simulink model "boostconverter_nap"  (R2016a)
settings: Solver=FixedStepDiscrete  SolverMode=SingleTasking  StartTime=0.0  StopTime=5e-5  FixedStep=5e-5  RelTol=1e-3
PreLoadFcn:
  | waijung.modelPreload; % Required for working with Waijung Blockset. Do not remove.
undefined symbols (not defined in the file): ARM, HSEOSC, Link, LQFP100, MDK, ST, STM32F407VE
libraries: stm32f4_adc_lib x1, stm32f4_device_config_lib x1, stm32f4_tim_lib x1
(part 3 of 3)

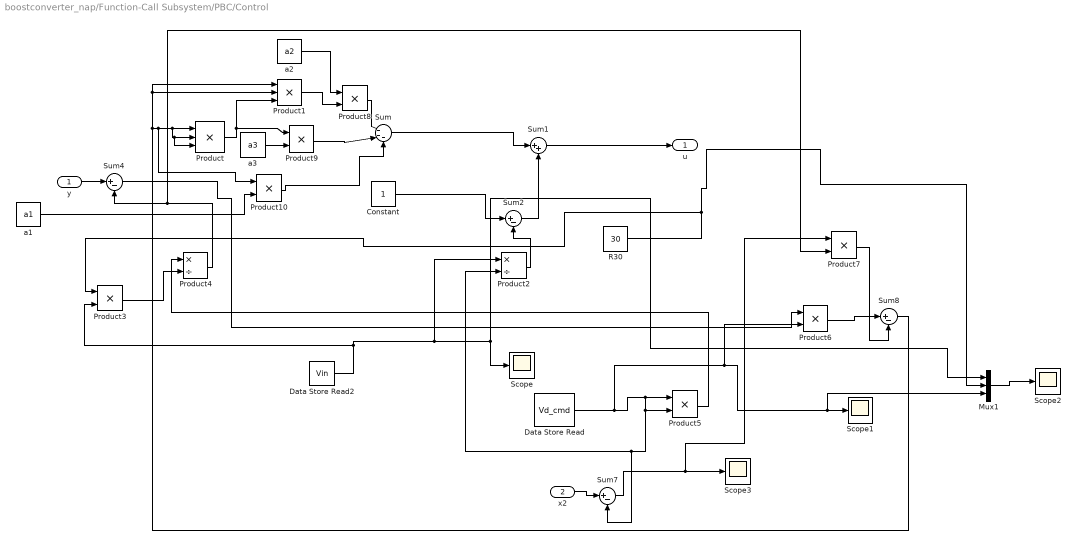
== system boostconverter_nap/Function-Call Subsystem/PBC/Control ==
  y : Inport
  x2 : Inport  Port=2
  Constant : Constant
  Data Store Read : DataStoreRead  DataStoreName=Vd_cmd
  Data Store Read2 : DataStoreRead  DataStoreName=Vin
  Mux1 : Mux  Inputs=3
  Product : Product  Inputs=3  RndMeth=Zero
  Product1 : Product  Inputs=3  RndMeth=Zero
  Product{3,5..7,9..10} (6 alike) : Product  RndMeth=Zero
  Product2 : Product  Inputs=*/  RndMeth=Zero
  Product4 : Product  Inputs=*/  RndMeth=Zero
  Product8 : Product
  "R30 " : Constant  Value=30
  Scope{,1..3} (4 alike) : Scope
  Sum : Sum  Inputs=|---
  Sum1 : Sum  Inputs=|++
  Sum{2,4,7..8} (4 alike) : Sum  Inputs=|+-
  a1 : DataStoreRead  DataStoreName=a1
  a2 : DataStoreRead  DataStoreName=a2
  a3 : DataStoreRead  DataStoreName=a3
  u : Outport
  wires:
  y/1 -> Sum4/1
  Product/1 -> Product9/1, Product1/3
  Product1/1 -> Product8/2
  Product10/1 -> Sum/3
  Product9/1 -> Sum/2
  Product8/1 -> Sum/1
  Constant/1 -> Sum2/1
  Product2/1 -> Sum2/2
  Sum2/1 -> Sum1/2
  Product3/1 -> Product4/2
  Product4/1 -> Product7/2, Sum4/2
  Data Store Read/1 -> Product5/2, Sum7/2, Product2/2, Product5/1, Product6/2, Mux1/3, Scope1/1
  Product5/1 -> Product4/1
  Data Store Read2/1 -> Product3/2, Product2/1, Mux1/1, Scope/1
  x2/1 -> Sum7/1
  Sum7/1 -> Product7/1, Scope3/1
  Sum4/1 -> Product6/1
  Product6/1 -> Sum8/1
  Product7/1 -> Sum8/2
  Sum8/1 -> Product1/2, Product1/1, Product10/1, Product/3, Product/2, Product/1
  Sum/1 -> Sum1/1
  "R30 "/1 -> Mux1/2, Product3/1
  Sum1/1 -> u/1
  a2/1 -> Product8/1
  a3/1 -> Product9/2
  a1/1 -> Product10/2
  Mux1/1 -> Scope2/1
